simulink model "dead_beat"  (R2018a)
settings: Solver=VariableStepAuto  StartTime=0.0  StopTime=10  RelTol=1e-3
settings Model: Creator=djoco  LastModifiedBy=djoco

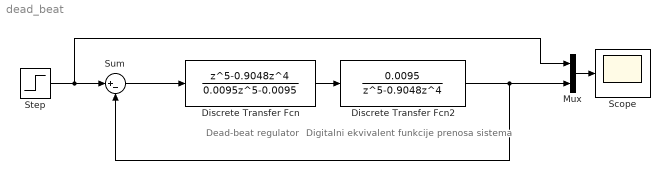
== system dead_beat ==
  note: Digitalni ekvivalent funkcije prenosa sistema
  note: Dead-beat regulator
  Discrete Transfer Fcn : DiscreteTransferFcn  Numerator=[1 -0.9048 0 0 0 0]  Denominator=[0.0095 0 0 0 0 -0.0095]  SampleTime=0.01
  Discrete Transfer Fcn2 : DiscreteTransferFcn  Numerator=[0.0095]  Denominator=[1 -0.9048 0 0 0 0]  SampleTime=0.01
  Mux : Mux  Inputs=2
  Scope : Scope
  Step : Step  SampleTime=0
  Sum : Sum  Inputs=|+-
  wires:
  Step/1 -> Mux/1, Sum/1
  Discrete Transfer Fcn2/1 -> Mux/2, Sum/2
  Sum/1 -> Discrete Transfer Fcn/1
  Mux/1 -> Scope/1
  Discrete Transfer Fcn/1 -> Discrete Transfer Fcn2/1
